simulink model "dspdltmd"  (Simulink 8.3)
settings: Solver=ode5  StartTime=0.0  StopTime=inf  RelTol=1e-3
libraries: dspwvfmcdlib x6, dsparch4 x1, simulink x1, dspmisc x1
settings Model: Creator=The MathWorks Inc.
settings OptimizationCC: BooleanDataType=off  ExpressionDepthLimit=2147483647  InitFltsAndDblsToZero=on
settings DebuggingCC: SaveWithParameterizedLinksMsg=none  SignalResolutionControl=TryResolveAllWithWarning  FcnCallInpInsideContextMsg=UseLocalSettings  StrictBusMsg=Warning
settings GRTTargetCC: TargetFcnLib=ansi_tfl_tmw.mat

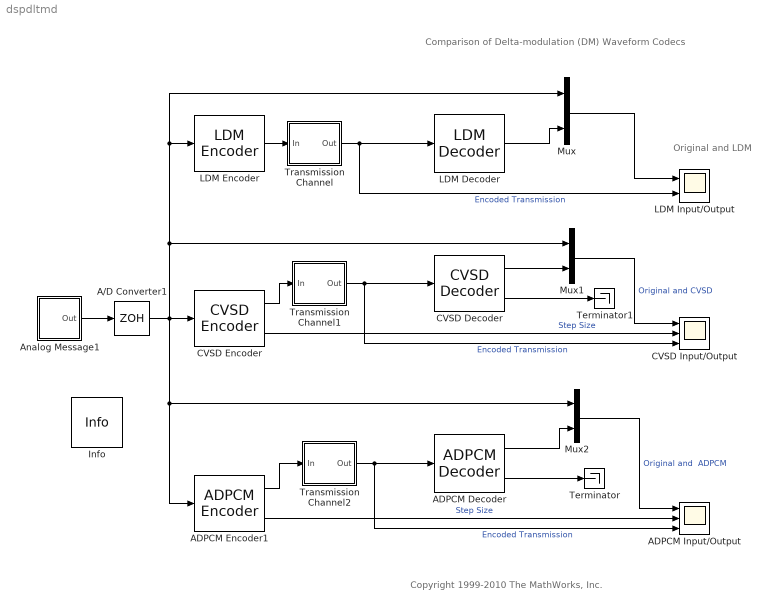
== system dspdltmd ==
  note: Original and LDM
  note: Comparison of Delta-modulation (DM) Waveform Codecs
  note: Copyright 1999-2010 The MathWorks, Inc.
  A/D Converter1 : ZeroOrderHold  SampleTime=1/8000
  ADPCM Decoder : dspwvfmcdlib/ADPCM Decoder  StepAttn=.5  StepGain=2  StepMax=0.5  StepMin=0.01  StepInit=0.1  AdpcmIntTau=0.99
  ADPCM Encoder1 : dspwvfmcdlib/ADPCM Encoder  EncStepAttn=.5  EncStepGain=2  EncStepMax=0.5  EncStepMin=0.01  EncStepInit=0.1  EncIntTau=0.99
  ADPCM Input/Output : Scope  NumInputPorts=3
      settings: TimeRange=0.02  YMin=-1.25~-0.75~-1.2  YMax=1.25~0.75~1.2  SaveName=ScopeData2
  Analog Message1 : Subsystem
  CVSD Decoder : dspwvfmcdlib/CVSD Decoder  DeltaMax=20  SylIntTau=0.99  DeltaMin=0.01  RecIntTau=0.96
  CVSD Encoder : dspwvfmcdlib/CVSD Encoder  EncDeltaMax=20  EncSylIntTau=0.99  EncDeltaMin=0.01  EncRecIntTau=0.96
  CVSD Input/Output : Scope  NumInputPorts=3
      settings: TimeRange=0.02  YMin=-1.25~-5~-0.1  YMax=1.25~5~1.1
  Info : dspmisc/Info  SystemSampleTime=-1
  LDM Decoder : dspwvfmcdlib/LDM Decoder  Tau=0.91
  LDM Encoder : dspwvfmcdlib/LDM Encoder  EncTau=0.91
  LDM Input/Output : Scope  NumInputPorts=2
      settings: TimeRange=0.02  YMin=-1.25~-0.1  YMax=1.25~1.1
  Mux : Mux  Inputs=2
  Mux1 : Mux  Inputs=2
  Mux2 : Mux  Inputs=2
  Terminator : Terminator
  Terminator1 : Terminator
  Transmission Channel : Subsystem
  Transmission Channel1 : Subsystem
  Transmission Channel2 : Subsystem
  wires:
  Mux/1 -> LDM Input/Output/1
  Transmission Channel/1(Out) -> LDM Decoder/1, LDM Input/Output/2  "Encoded Transmission"
  LDM Decoder/1 -> Mux/2
  LDM Encoder/1 -> Transmission Channel/1(In)
  Mux1/1 -> CVSD Input/Output/1  "Original and CVSD"
  Transmission Channel1/1(Out) -> CVSD Decoder/1, CVSD Input/Output/3  "Encoded Transmission"
  Analog Message1/1(Out) -> A/D Converter1/1
  CVSD Decoder/1 -> Mux1/2
  CVSD Encoder/1 -> Transmission Channel1/1(In)
  CVSD Encoder/2 -> CVSD Input/Output/2  "Step Size"
  A/D Converter1/1 -> CVSD Encoder/1, Mux1/1, LDM Encoder/1, Mux/1, ADPCM Encoder1/1, Mux2/1
  Mux2/1 -> ADPCM Input/Output/1  "Original and  ADPCM"
  Transmission Channel2/1(Out) -> ADPCM Decoder/1, ADPCM Input/Output/3  "Encoded Transmission"
  ADPCM Decoder/1 -> Mux2/2
  ADPCM Encoder1/1 -> Transmission Channel2/1(In)
  ADPCM Encoder1/2 -> ADPCM Input/Output/2  "Step Size"
  ADPCM Decoder/2 -> Terminator/1
  CVSD Decoder/2 -> Terminator1/1

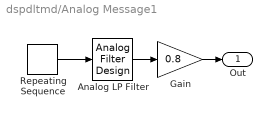
== system dspdltmd/Analog Message1 ==
  Analog LP Filter : dsparch4/Analog Filter Design  method=Butterworth  filttype=Lowpass  N=5  Wlo=2*pi*400  Whi=80  Rp=3  Rs=40
  Gain : Gain  Gain=0.8  SaturateOnIntegerOverflow=on  OutDataTypeStr=Inherit: Same as input  ParamDataTypeStr=Inherit: Same as input
  Repeating Sequence : simulink/Sources/Repeating Sequence  rep_seq_t=[ 0 0.005 0.005+eps(0.005) 0.015 0.015+eps(0.015) 0.02]  rep_seq_y=[ 1 1 -1+0*eps(0.005) -1 1+0*eps(0.015) 1]
  Out : Outport
  wires:
  Analog LP Filter/1 -> Gain/1
  Repeating Sequence/1 -> Analog LP Filter/1
  Gain/1 -> Out/1

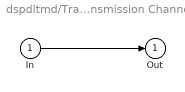
== system dspdltmd/Transmission Channel ==
  In : Inport
  Out : Outport
  wires:
  In/1 -> Out/1

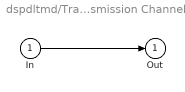
== system dspdltmd/Transmission Channel1 ==
  In : Inport
  Out : Outport
  wires:
  In/1 -> Out/1

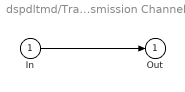
== system dspdltmd/Transmission Channel2 ==
  In : Inport
  Out : Outport
  wires:
  In/1 -> Out/1
